simulink model "SmallManufacturingSystem"  (Simulink 7.9)
settings: Solver=FixedStepDiscrete  StartTime=0.0  StopTime=1000  RelTol=1e-3
undefined symbols (not defined in the file): des, gcbh
settings Model: Creator=tsprock3  LastModifiedBy=tsprock3
settings SimEventsCC: propDiagAttribOutput=1  propDiagFcnCallOutput=1

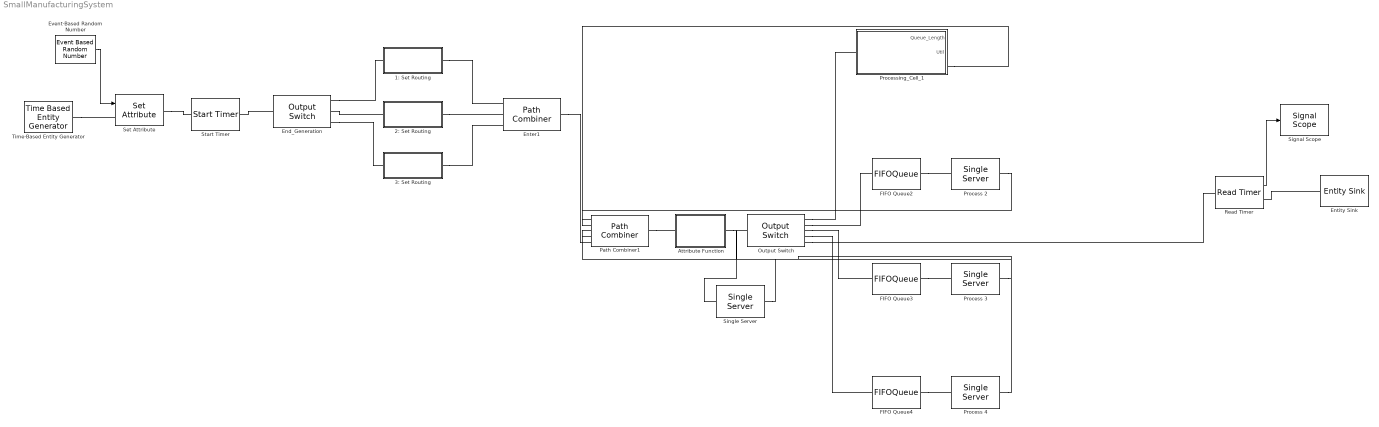
== system SmallManufacturingSystem ==
  "1: Set Routing " : Subsystem
  2: Set Routing : Subsystem
  3: Set Routing : Subsystem
  Attribute Function : Subsystem  LoadFcn=des.afb.attributefunction_support(gcb,'LoadFcn');  StartFcn=des.afb.attributefunction_support(gcb,'StartFcn');  mask(Attribute Function){OutputNamePrefix=out_}
      mask prompts: OutputNamePrefix "Prefix name"
      settings: CopyFcn=des.afb.attributefunction_support(gcb,'CopyFcn');  OpenFcn=des.afb.attributefunction_support(gcb,'OpenFcn');  ErrorFcn=des.afb.error_redirect
      mask Help: slhelp(gcbh)
      mask Display: image(des_iconLoad('attribFunction.jpg'),'center');
  End_Generation : OutputSwitch  SwitchingCriterion=From attribute  AttributeName=Part_Type
  Enter1 : PathCombiner
  Entity Sink : EntitySink
  Event-Based Random Number : EventBasedRandomNumber  Distribution=Arbitrary discrete  valueVecDisc=[1 2 3]  probVecDisc=[0.26 .48 .26]  Seed=33601
  FIFO Queue2 : FIFOQueue
  FIFO Queue3 : FIFOQueue
  FIFO Queue4 : FIFOQueue
  Output Switch : OutputSwitch  NumberOutputPorts=5  SwitchingCriterion=Equiprobable  AttributeName=Destination
  Path Combiner1 : PathCombiner  NumberInputPorts=5
  Process 2 : SingleServer  ServiceTimeFrom=Attribute  AttributeName=ServiceTime2
  Process 3 : SingleServer  ServiceTimeFrom=Attribute  AttributeName=ServiceTime3
  Process 4 : SingleServer  ServiceTimeFrom=Attribute  AttributeName=ServiceTime4
  Processing_Cell_1 : Subsystem
  Read Timer : ReadTimer  StatAverageTimeElapsed=on
      settings: OutputPortMap=o3
  Set Attribute : SetAttribute  AttributeName=Part_Type  AttributeFrom=Signal port  EvaluatedAttributeValue={[]}
  Signal Scope : SignalScope  LoadFcn=des.scope.CallbackSupport('seLoadFcn',gcbh)  StartFcn=des.scope.CallbackSupport('seStartFcn',gcbh)  StopFcn=des.scope.CallbackSupport('seStopFcn',gcbh)
      settings: CopyFcn=des.scope.CallbackSupport('seCopyFcn',gcbh)  DeleteFcn=des.scope.CallbackSupport('seDeleteFcn',gcbh)  PreSaveFcn=des.scope.CallbackSupport('sePreSaveFcn',gcbh)  NameChangeFcn=des.scope.CallbackSupport('seNameChangeFcn',gcbh)  OpenFcn=des.scope.CallbackSupport('seOpenFcn',gcbh)
  Single Server : SingleServer  ServiceTime=0
  Start Timer : StartTimer
  Time-Based Entity Generator : TimeBasedEntityGenerator  Distribution=Exponential  InitialSeed=36818  Maximum=5  Mean=13
  wires:
  Event-Based Random Number/1 -> Set Attribute/1
  Read Timer/1 -> Signal Scope/1
  connections:
  Time-Based Entity Generator/RConn1 -- Set Attribute/LConn1
  Set Attribute/RConn1 -- Start Timer/LConn1
  FIFO Queue2/RConn1 -- Process 2/LConn1
  FIFO Queue3/RConn1 -- Process 3/LConn1
  FIFO Queue4/RConn1 -- Process 4/LConn1
  Read Timer/RConn1 -- Entity Sink/LConn1
  Start Timer/RConn1 -- End_Generation/LConn1
  End_Generation/RConn1 -- "1: Set Routing "/RConn1
  End_Generation/RConn2 -- 2: Set Routing/RConn1
  End_Generation/RConn3 -- 3: Set Routing/RConn1
  "1: Set Routing "/LConn1 -- Enter1/LConn1
  2: Set Routing/LConn1 -- Enter1/LConn2
  3: Set Routing/LConn1 -- Enter1/LConn3
  Path Combiner1/RConn1 -- Attribute Function/LConn1
  Output Switch/RConn1 -- Processing_Cell_1/LConn1
  Output Switch/RConn2 -- FIFO Queue2/LConn1
  Output Switch/RConn3 -- FIFO Queue3/LConn1
  Output Switch/RConn4 -- FIFO Queue4/LConn1
  Processing_Cell_1/RConn1 -- Path Combiner1/LConn1
  Process 2/RConn1 -- Path Combiner1/LConn2
  Process 3/RConn1 -- Path Combiner1/LConn3
  Process 4/RConn1 -- Path Combiner1/LConn4
  Enter1/RConn1 -- Path Combiner1/LConn5
  Output Switch/RConn5 -- Read Timer/LConn1
  Attribute Function/RConn1 -- Single Server/LConn1
  Single Server/RConn1 -- Output Switch/LConn1

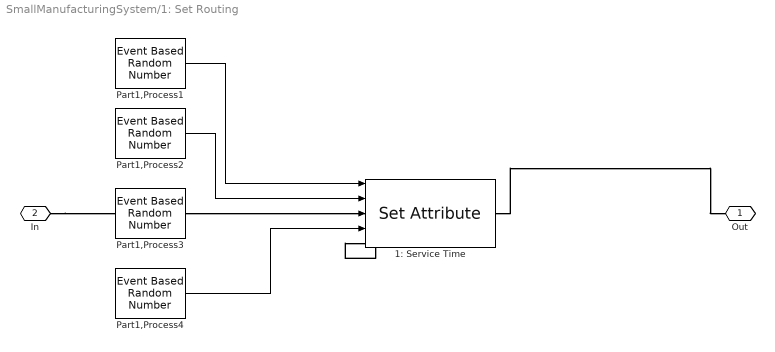
== system SmallManufacturingSystem/1: Set Routing  ==
  1: Service Time : SetAttribute  AttributeName=ServiceTime1|ServiceTime2|ServiceTime3|ServiceTime4|Route|Destination  AttributeFrom=Signal port|Signal port|Signal port|Signal port|Dialog|Dialog  AttributeValue=1|1|1|1|[1 2 3 4 5 5].'|1  AttributeTreatAsVector=1|1|1|1|0|1  EvaluatedAttributeValue={[];[];[];[];[1 2 3 4 5 5].';1}
      settings: InputPortMap=u0,u1,u2,u3
  Part1,Process1 : EventBasedRandomNumber  Distribution=Triangular  minTri=6  maxTri=10  modeTri=8  Seed=60161
  Part1,Process2 : EventBasedRandomNumber  Distribution=Triangular  minTri=6  maxTri=10  modeTri=8  Seed=63378
  Part1,Process3 : EventBasedRandomNumber  Distribution=Triangular  minTri=15  maxTri=25  modeTri=20  Seed=1059
  Part1,Process4 : EventBasedRandomNumber  Distribution=Triangular  minTri=8  maxTri=16  modeTri=12  Seed=4276
  Out : PMIOPort  Port=1  Side=Left
  In : PMIOPort  Port=2  Side=Right
  wires:
  Part1,Process1/1 -> 1: Service Time/1
  Part1,Process2/1 -> 1: Service Time/2
  Part1,Process3/1 -> 1: Service Time/3
  Part1,Process4/1 -> 1: Service Time/4
  connections:
  1: Service Time/RConn1 -- Out/RConn1
  In/RConn1 -- 1: Service Time/LConn1

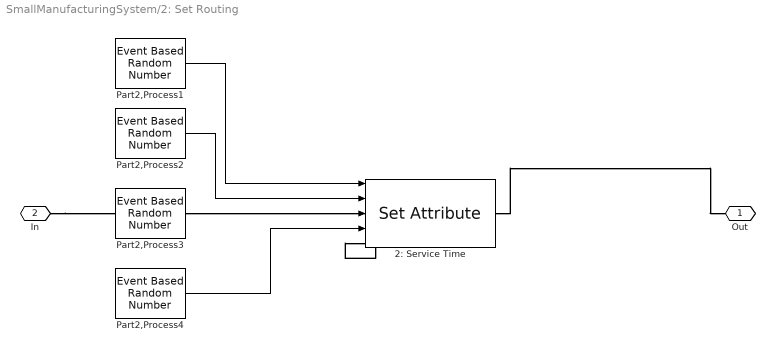
== system SmallManufacturingSystem/2: Set Routing ==
  2: Service Time : SetAttribute  AttributeName=ServiceTime1|ServiceTime2|ServiceTime3|ServiceTime4|Route|Destination  AttributeFrom=Signal port|Signal port|Signal port|Signal port|Dialog|Dialog  AttributeValue=1|1|1|1|[1 2 4 2 3 5].'|1  AttributeTreatAsVector=1|1|1|1|0|1  EvaluatedAttributeValue={[];[];[];[];[1 2 4 2 3 5].';1}
      settings: InputPortMap=u0,u1,u2,u3
  Part2,Process1 : EventBasedRandomNumber  Distribution=Triangular  minTri=11  maxTri=15  modeTri=13  Seed=7493
  Part2,Process2 : EventBasedRandomNumber  Distribution=Triangular  minTri=4  maxTri=8  modeTri=6  Seed=10710
  Part2,Process3 : EventBasedRandomNumber  Distribution=Triangular  minTri=27  maxTri=39  modeTri=33  Seed=13927
  Part2,Process4 : EventBasedRandomNumber  Distribution=Triangular  minTri=15  maxTri=21  modeTri=18  Seed=17144
  Out : PMIOPort  Port=1  Side=Left
  In : PMIOPort  Port=2  Side=Right
  wires:
  Part2,Process1/1 -> 2: Service Time/1
  Part2,Process2/1 -> 2: Service Time/2
  Part2,Process3/1 -> 2: Service Time/3
  Part2,Process4/1 -> 2: Service Time/4
  connections:
  2: Service Time/RConn1 -- Out/RConn1
  In/RConn1 -- 2: Service Time/LConn1

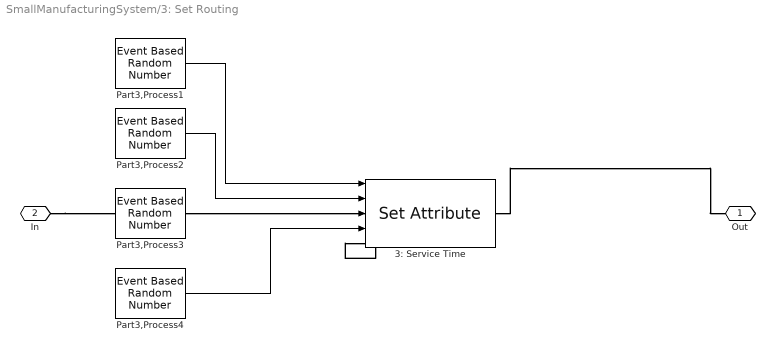
== system SmallManufacturingSystem/3: Set Routing ==
  3: Service Time : SetAttribute  AttributeName=ServiceTime1|ServiceTime2|ServiceTime3|ServiceTime4|Route|Destination  AttributeFrom=Signal port|Signal port|Signal port|Signal port|Dialog|Dialog  AttributeValue=1|1|1|1|[2 1 3 5 5 5].'|2  AttributeTreatAsVector=1|1|1|1|0|1  EvaluatedAttributeValue={[];[];[];[];[2 1 3 5 5 5].';2}
      settings: InputPortMap=u0,u1,u2,u3
  Part3,Process1 : EventBasedRandomNumber  Distribution=Triangular  minTri=7  maxTri=13  modeTri=10  Seed=20361
  Part3,Process2 : EventBasedRandomNumber  Distribution=Triangular  minTri=7  maxTri=11  modeTri=9  Seed=23578
  Part3,Process3 : EventBasedRandomNumber  Distribution=Triangular  minTri=18  maxTri=28  modeTri=23  Seed=26795
  Part3,Process4 : EventBasedRandomNumber  Distribution=Triangular  minTri=8  maxTri=16  modeTri=12  Seed=30384
  Out : PMIOPort  Port=1  Side=Left
  In : PMIOPort  Port=2  Side=Right
  wires:
  Part3,Process1/1 -> 3: Service Time/1
  Part3,Process2/1 -> 3: Service Time/2
  Part3,Process3/1 -> 3: Service Time/3
  Part3,Process4/1 -> 3: Service Time/4
  connections:
  3: Service Time/RConn1 -- Out/RConn1
  In/RConn1 -- 3: Service Time/LConn1

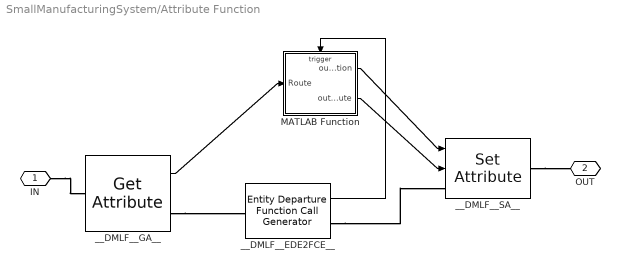
== system SmallManufacturingSystem/Attribute Function ==
  MATLAB Function : MATLAB Function  TreatAsAtomicUnit=on
  __DMLF__EDE2FCE__ : EntityDepartureFunctionCallGenerator
  __DMLF__GA__ : GetAttribute  AttributeName=Route  AttributeSendTiming=Before entity departure  EvaluatedDefaultAttributeValue={[]}  IsInsideAFB=on
      settings: OutputPortMap=o1
  __DMLF__SA__ : SetAttribute  AttributeName=Destination|Route  AttributeFrom=Signal port|Signal port  AttributeValue=1|1  AttributeTreatAsVector=1|1  EvaluatedAttributeValue={[];[]}  IsInsideAFB=on
      settings: InputPortMap=u0,u1
  IN : PMIOPort  Port=1  Side=Left
  OUT : PMIOPort  Port=2  Side=Right
  wires:
  __DMLF__EDE2FCE__/1 -> MATLAB Function/Trigger
  __DMLF__GA__/1 -> MATLAB Function/1(Route)
  MATLAB Function/1(out_Destination) -> __DMLF__SA__/1
  MATLAB Function/2(out_Route) -> __DMLF__SA__/2
  connections:
  __DMLF__EDE2FCE__/RConn1 -- __DMLF__SA__/LConn1
  __DMLF__GA__/RConn1 -- __DMLF__EDE2FCE__/LConn1
  IN/RConn1 -- __DMLF__GA__/LConn1
  __DMLF__SA__/RConn1 -- OUT/RConn1

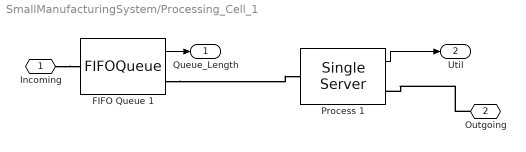
== system SmallManufacturingSystem/Processing_Cell_1 ==
  "FIFO Queue 1 " : FIFOQueue  StatAverageQueueLength=on
      settings: OutputPortMap=o3
  Process 1 : SingleServer  ServiceTimeFrom=Attribute  AttributeName=ServiceTime1  StatUtilization=on
      settings: OutputPortMap=o5
  Incoming : PMIOPort  Port=1  Side=Left
  Outgoing : PMIOPort  Port=2  Side=Right
  Queue_Length : Outport
  Util : Outport  Port=2
  wires:
  "FIFO Queue 1 "/1 -> Queue_Length/1
  Process 1/1 -> Util/1
  connections:
  "FIFO Queue 1 "/RConn1 -- Process 1/LConn1
  Incoming/RConn1 -- "FIFO Queue 1 "/LConn1
  Outgoing/RConn1 -- Process 1/RConn1

== matlab function Attribute Function/MATLAB Function ==
  data: Route input double; out_Destination output double; out_Route output double
  events: trigger input FUNCTION_CALL_EVENT
function [out_Destination, out_Route] = fcn(Route)
%FCN    Access and modify attributes with MATLAB 
% 
% Input arguments must match the attribute names.
% Output arguments must be out_<AttributeName>,
% e.g., out_ServiceTime where ServiceTime is the attribute name.
% 
% The output attribute will be created if it is not present.
%

out_Destination = Route(1);
out_Route = Route([2:end 1]);
